simulink model "model5_2f"  (R2024b)
settings: Solver=VariableStepAuto  StartTime=0.0  StopTime=10  MaxStep=1e-3  RelTol=1e-3
values from neighbouring files (symbols this model uses):
  dx0 = 5    [model5_params.m]    (also in problem_2c.m = sqrt(2/m*(Esys-m*g*y0)); problem_2d.m = sqrt(2/m*(Esys-m*g*y0)); problem_2e.m)
  dy0 = 0    [model5_params.m]    (also in problem_2c.m; problem_2d.m; problem_2e.m)
  g = 9.81    [model5_params.m]    (also in problem_2c.m; problem_2d.m; problem_2e.m)
  k = 20000    [model5_params.m]    (also in problem_2c.m; problem_2d.m; problem_2e.m)
  l0 = 1    [model5_params.m]    (also in problem_2c.m; problem_2d.m; problem_2e.m)
  m = 80    [model5_params.m]    (also in problem_2c.m; problem_2d.m; problem_2e.m)
  model_version = model    [problem_2c.m]    (also in problem_2d.m)
  noise_gain = noise_gains(gain_idx)    [problem_2e.m]
  noise_seed = noise_seed + 1    (= 1)    [problem_2e.m]
  polys = [2.34748450027  -0.232659696524  0.683870176359  1.04028141255; 1.40200554185  0.146392538734  0.650336688357  1.17942827023; 6.90999581965  -3.82728362568  1.71997695345  0.733552254583]    [polys.mat]    (also in problem_2d.m = NaN(3,4))
  x0 = []    [ipm_animation2.m]    (also in model5_params.m = 0; problem_2c.m = 0; problem_2d.m = 0; problem_2e.m = 0)
  y0 = 1    [model5_params.m]    (also in problem_2c.m = y0Vec(y0Idx); problem_2d.m = y0Vec(y0Idx); problem_2e.m)
libraries: simulink_extras x1
settings Model: Creator=hgeyer  LastModifiedBy=gnastacast

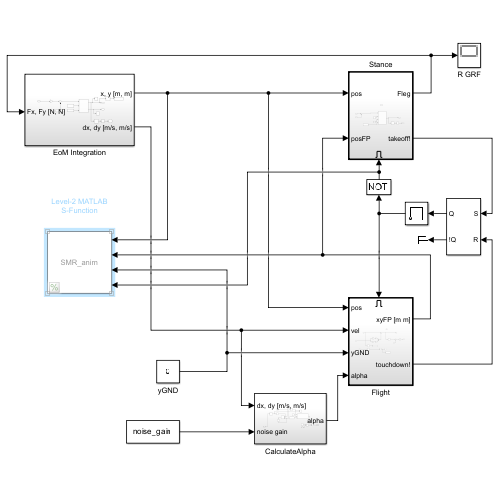
[thumbnail: Simulink's stored preview of the top-level diagram]
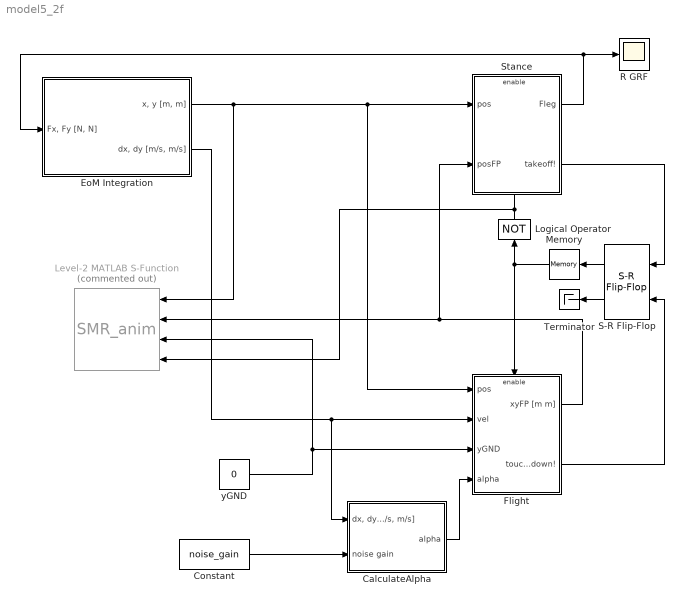
== system model5_2f ==
  CalculateAlpha : Subsystem
  Constant : Constant  Value=noise_gain
  EoM Integration : Subsystem
  Flight : Subsystem
  Level-2 MATLAB S-Function : M-S-Function  Commented=on  FunctionName=SMR_anim  Parameters=0.01
  Logical Operator : Logic  Operator=NOT  AllPortsSameDT=off  OutDataTypeStr=boolean
  Memory : Memory  InitialCondition=1
  R GRF : Scope
  S-R Flip-Flop : simulink_extras/Flip Flops/S-R Flip-Flop  initial_condition=1
  Stance : Subsystem
  Terminator : Terminator
  yGND : Constant  Value=0
  wires:
  EoM Integration/1("x, y [m, m]") -> Level-2 MATLAB S-Function/1, Flight/1(pos), Stance/1(pos)
  Stance/2(takeoff!) -> S-R Flip-Flop/1
  Flight/2(touchdown!) -> S-R Flip-Flop/2
  S-R Flip-Flop/1 -> Memory/1
  Memory/1 -> Flight/Enable, Logical Operator/1
  S-R Flip-Flop/2 -> Terminator/1
  Flight/1(xyFP [m m]) -> Level-2 MATLAB S-Function/2, Stance/2(posFP)
  Stance/1(Fleg) -> R GRF/1, EoM Integration/1("Fx, Fy [N, N]")
  yGND/1 -> Level-2 MATLAB S-Function/3, Flight/3(yGND)
  Logical Operator/1 -> Level-2 MATLAB S-Function/4, Stance/Enable
  EoM Integration/2("dx, dy [m/s, m/s]") -> Flight/2(vel), CalculateAlpha/1("dx, dy [m/s, m/s]")
  CalculateAlpha/1(alpha) -> Flight/4(alpha)
  Constant/1 -> CalculateAlpha/2(noise gain)

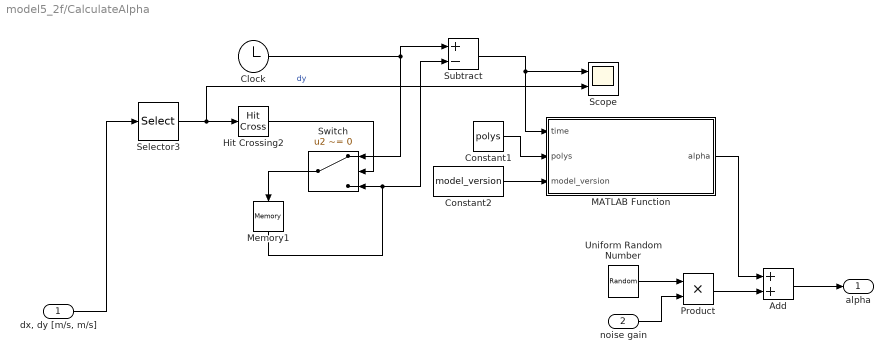
== system model5_2f/CalculateAlpha ==
  "dx, dy [m/s, m/s]" : Inport
  noise gain : Inport  Port=2
  Add : Sum
  Clock : Clock
  Constant1 : Constant  Value=polys
  Constant2 : Constant  Value=model_version
  Hit Crossing2 : HitCross  HitCrossingOffset=eps  HitCrossingDirection=falling
  MATLAB Function : MATLAB Function  TreatAsAtomicUnit=on
  Memory1 : Memory
  Product : Product
  Scope : Scope  NumInputPorts=2
  Selector3 : Selector  InputPortWidth=2  IndexOptions=Index vector (dialog)  Indices=2  OutputSizes=1
  Subtract : Sum  Inputs=+-
  Switch : Switch  Criteria=u2 ~= 0  SaturateOnIntegerOverflow=off  InputSameDT=off
  Uniform Random Number : UniformRandomNumber  Seed=noise_seed  SampleTime=0.1
  alpha : Outport
  wires:
  Memory1/1 -> Subtract/2, Switch/3
  MATLAB Function/1(alpha) -> Add/1
  Selector3/1 -> Scope/2, Hit Crossing2/1  "dy"
  Constant2/1 -> MATLAB Function/3(model_version)
  Hit Crossing2/1 -> Switch/2
  Subtract/1 -> MATLAB Function/1(time), Scope/1
  Clock/1 -> Subtract/1, Switch/1
  Switch/1 -> Memory1/1
  Constant1/1 -> MATLAB Function/2(polys)
  "dx, dy [m/s, m/s]"/1 -> Selector3/1
  Uniform Random Number/1 -> Product/1
  noise gain/1 -> Product/2
  Add/1 -> alpha/1
  Product/1 -> Add/2

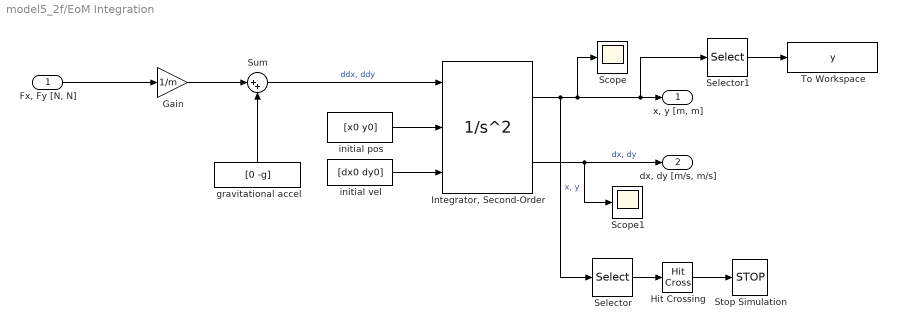
== system model5_2f/EoM Integration ==
  "Fx, Fy [N, N]" : Inport
  Gain : Gain  Gain=1/m
  Hit Crossing : HitCross  HitCrossingDirection=falling
  "Integrator, Second-Order" : SecondOrderIntegrator  ICSourceX=external  ICSourceDXDT=external
  Scope : Scope
  Scope1 : Scope
  Selector : Selector  InputPortWidth=2  IndexOptions=Index vector (dialog)  Indices=2  OutputSizes=1
  Selector1 : Selector  InputPortWidth=2  IndexOptions=Index vector (dialog)  Indices=2  OutputSizes=1
  Stop Simulation : Stop
  Sum : Sum  Inputs=|++
  To Workspace : ToWorkspace  VariableName=y  SaveFormat=Structure  SampleTime=-1
      settings: Save2DSignal=2-D array (concatenate along first dimension)
  gravitational accel : Constant  Value=[0 -g]
  initial pos : Constant  Value=[x0 y0]
  initial vel : Constant  Value=[dx0 dy0]
  "x, y [m, m]" : Outport
  "dx, dy [m/s, m/s]" : Outport  Port=2
  wires:
  "Integrator, Second-Order"/2 -> Scope1/1, "dx, dy [m/s, m/s]"/1  "dx, dy"
  Sum/1 -> "Integrator, Second-Order"/1  "ddx, ddy"
  initial pos/1 -> "Integrator, Second-Order"/2
  Gain/1 -> Sum/1
  gravitational accel/1 -> Sum/2
  "Integrator, Second-Order"/1 -> Scope/1, Selector1/1, "x, y [m, m]"/1, Selector/1  "x, y"
  initial vel/1 -> "Integrator, Second-Order"/3
  "Fx, Fy [N, N]"/1 -> Gain/1
  Selector/1 -> Hit Crossing/1
  Hit Crossing/1 -> Stop Simulation/1
  Selector1/1 -> To Workspace/1

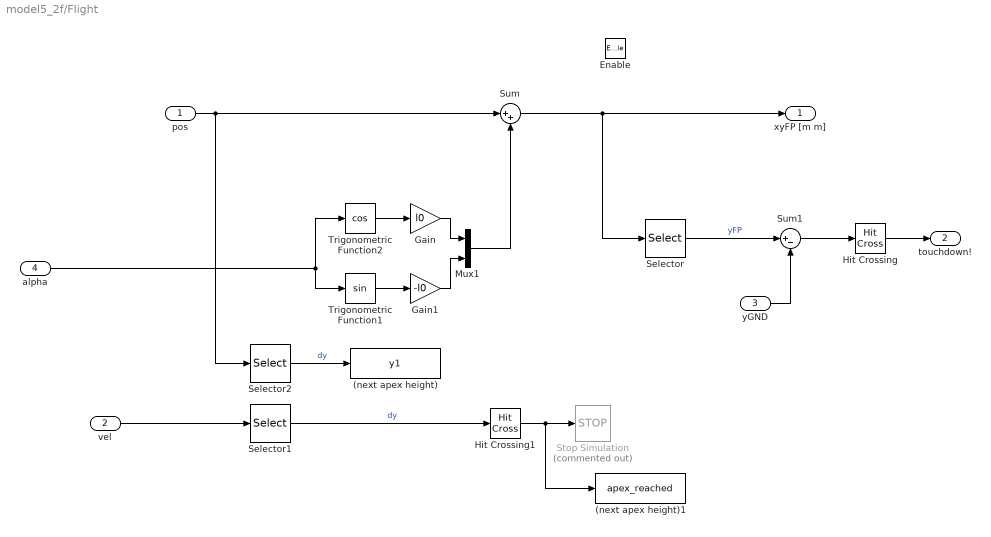
== system model5_2f/Flight ==
  pos : Inport
  vel : Inport  Port=2
  yGND : Inport  Port=3
  alpha : Inport  Port=4
  Enable : EnablePort  StatesWhenEnabling=reset
      settings: AttributesFormatString=when enabled: %<StatesWhenEnabling>
  (next apex height) : ToWorkspace  VariableName=y1  SampleTime=-1
      settings: MaxDataPoints=1
  (next apex height)1 : ToWorkspace  VariableName=apex_reached  SampleTime=-1
      settings: MaxDataPoints=1
  Gain : Gain  Gain=l0
  Gain1 : Gain  Gain=-l0
  Hit Crossing : HitCross  HitCrossingDirection=falling
  Hit Crossing1 : HitCross  HitCrossingOffset=eps  HitCrossingDirection=falling
  Mux1 : Mux  Inputs=2
  Selector : Selector  InputPortWidth=2  IndexOptions=Index vector (dialog)  Indices=2  OutputSizes=1
  Selector1 : Selector  InputPortWidth=2  IndexOptions=Index vector (dialog)  Indices=2  OutputSizes=1
  Selector2 : Selector  InputPortWidth=2  IndexOptions=Index vector (dialog)  Indices=2  OutputSizes=1
  Stop Simulation : Stop  Commented=on
  Sum : Sum  Inputs=|++
  Sum1 : Sum  Inputs=|+-
  Trigonometric Function1 : Trigonometry
  Trigonometric Function2 : Trigonometry  Operator=cos
  xyFP [m m] : Outport  InitialOutput=0
      settings: AttributesFormatString=|
      | when disabled: %<OutputWhenDisabled>
      | initial: %<InitialOutput>
  touchdown! : Outport  Port=2  OutputWhenDisabled=reset  InitialOutput=0
      settings: AttributesFormatString=|
      | when disabled: %<OutputWhenDisabled>
      | initial: %<InitialOutput>
  wires:
  Hit Crossing/1 -> touchdown!/1
  Sum1/1 -> Hit Crossing/1
  yGND/1 -> Sum1/2
  alpha/1 -> Trigonometric Function2/1, Trigonometric Function1/1
  Trigonometric Function2/1 -> Gain/1
  Trigonometric Function1/1 -> Gain1/1
  Gain/1 -> Mux1/1
  Gain1/1 -> Mux1/2
  pos/1 -> Selector2/1, Sum/1
  Mux1/1 -> Sum/2
  Sum/1 -> Selector/1, xyFP [m m]/1
  Selector/1 -> Sum1/1  "yFP"
  vel/1 -> Selector1/1
  Selector1/1 -> Hit Crossing1/1  "dy"
  Hit Crossing1/1 -> (next apex height)1/1, Stop Simulation/1
  Selector2/1 -> (next apex height)/1  "dy"

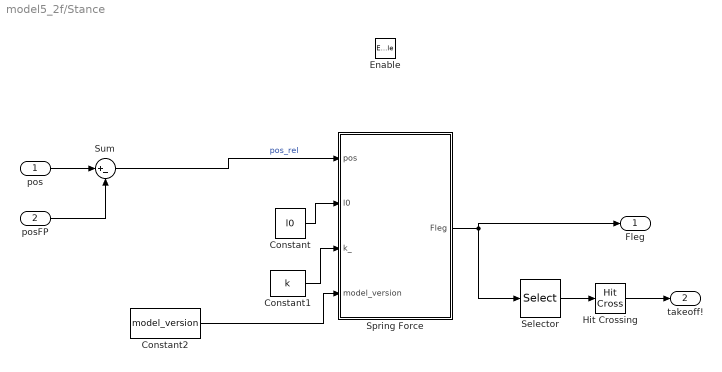
== system model5_2f/Stance ==
  pos : Inport
  posFP : Inport  Port=2
  Enable : EnablePort  StatesWhenEnabling=reset
      settings: AttributesFormatString=when enabled: %<StatesWhenEnabling>
  Constant : Constant  Value=l0
  Constant1 : Constant  Value=k
  Constant2 : Constant  Value=model_version
  Hit Crossing : HitCross  HitCrossingDirection=falling
  Selector : Selector  InputPortWidth=2  IndexOptions=Index vector (dialog)  Indices=2  OutputSizes=1
  Spring Force : MATLAB Function  TreatAsAtomicUnit=on
  Sum : Sum  Inputs=|+-
  Fleg : Outport  OutputWhenDisabled=reset  InitialOutput=[0; 0]
      settings: AttributesFormatString=|
      | when disabled: %<OutputWhenDisabled>
      | initial: %<InitialOutput>
  takeoff! : Outport  Port=2  OutputWhenDisabled=reset  InitialOutput=0
      settings: AttributesFormatString=|
      | when disabled: %<OutputWhenDisabled>
      | initial: %<InitialOutput>
  wires:
  Spring Force/1(Fleg) -> Fleg/1, Selector/1
  pos/1 -> Sum/1
  posFP/1 -> Sum/2
  Sum/1 -> Spring Force/1(pos)  "pos_rel"
  Hit Crossing/1 -> takeoff!/1
  Constant/1 -> Spring Force/2(l0)
  Constant1/1 -> Spring Force/3(k_)
  Selector/1 -> Hit Crossing/1
  Constant2/1 -> Spring Force/4(model_version)

== matlab function model5_2f/CalculateAlpha/MATLAB Function ==
  data: time input; polys input; alpha output; model_version input
function alpha = fcn(time, polys, model_version)

alpha = polyval(polys(model_version,:), time);

== matlab function model5_2f/Stance/Spring Force ==
  data: pos input; Fleg output; l0 input; k_ input; model_version input
function Fleg  = fcn(pos, l0, k_, model_version)

l = sqrt(pos(1)^2 + pos(2)^2);
k = k_;
switch model_version
    case 1
        k = k_;
    case 2
        k = k_*2;
    case 3
        if (l/l0) < 0.95
            k = k_/2;
        end
    otherwise
        error('Undefined model version')
end

Fs = k * (l0 - l);

Fleg = Fs / l * pos;
